simulink model "noControlObserver"  (R2015a)
settings: Solver=ode45  StartTime=0.0  StopTime=tijd  RelTol=1e-3
values from neighbouring files (symbols this model uses):
  A2 = A    [LQControl.m]    (also in LQControl_script.m)
  AS = A2-H*C2    [LQControl.m]    (also in LQControl_script.m)
  B2 = B    [LQControl.m]    (also in LQControl_script.m)
  BS = [H B2-H*D2]    [LQControl.m]    (also in LQControl_script.m)
  C2 = [0.5 0.4 0 ... (first row only)    [LQControl.m]    (also in LQControl_script.m)
  CS = [1 0 0 ... (first row only)    [LQControl.m]    (also in LQControl_script.m)
  D2 = [0;0]    [LQControl.m]    (also in LQControl_script.m)
  DS = [0 0 0 ... (first row only)    [LQControl.m]    (also in LQControl_script.m)
  k0 = -1.22*10^3    (= -1220)    [LQControl.m]    (also in LQControl_script.m)
  kev = (Y*a*kV)/(d1 - b1 + Y*a)    (= 2222.22222222)    [LQControl.m]    (also in LQControl_script.m)
  kin = 0    [LQControl.m]    (also in LQControl_script.m)
  s0 = 500    [LQControl.m]    (also in LQControl_script.m)
  v0 = -2.22    [LQControl.m]    (also in LQControl_script.m)
  vev = (a*kV*(b1 - d1))/(d3*(d1 - b1 + Y*a))    (= 22.2222222222)    [LQControl.m]    (also in LQControl_script.m)
settings Model: Creator=Ward  LastModifiedBy=Ward

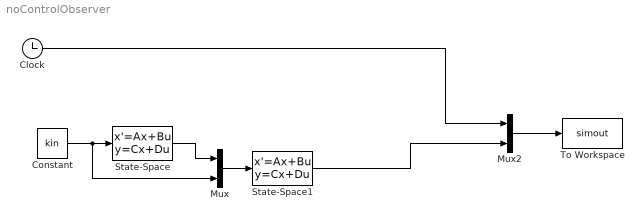
== system noControlObserver ==
  Clock : Clock
  Constant : Constant  Value=kin
  Mux : Mux  Inputs=2
  Mux2 : Mux  Inputs=2
  State-Space : StateSpace  A=A2  B=B2  C=C2  D=D2  X0=[k0-kev;s0;v0-vev]
  State-Space1 : StateSpace  A=AS  B=BS  C=CS  D=DS  X0=[0;0;0]
  To Workspace : ToWorkspace  VariableName=simout  SampleTime=-1
  wires:
  Constant/1 -> Mux/2, State-Space/1
  Clock/1 -> Mux2/1
  Mux2/1 -> To Workspace/1
  Mux/1 -> State-Space1/1
  State-Space/1 -> Mux/1
  State-Space1/1 -> Mux2/2
